simulink model "LorenzModel_book_example"  (R2023a)
settings: Solver=VariableStepAuto  StartTime=0.0  StopTime=50  RelTol=1e-3
settings Model: Creator=axobj  LastModifiedBy=axobj

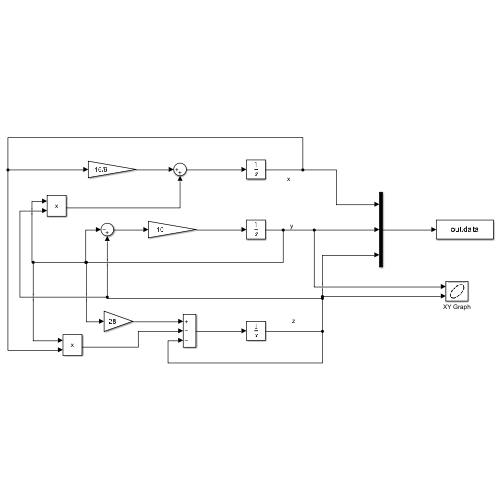
[thumbnail: Simulink's stored preview of the top-level diagram]
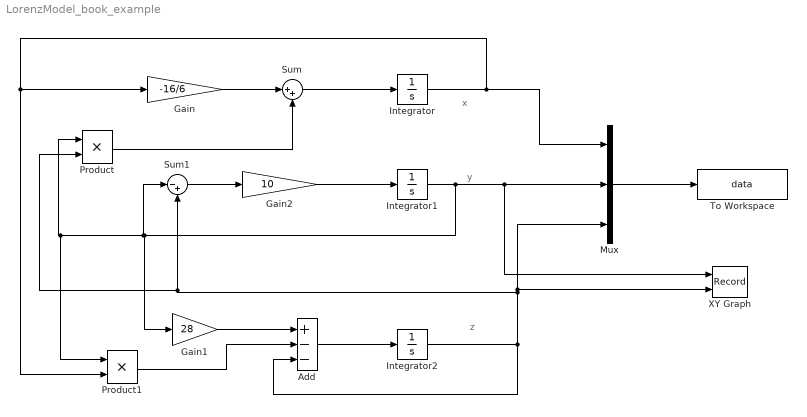
== system LorenzModel_book_example ==
  note: x
  note: y
  note: z
  Add : Sum  Inputs=+--
  Gain : Gain  Gain=-16/6
  Gain1 : Gain  Gain=28
  Gain2 : Gain  Gain=10
  Integrator : Integrator  InitialCondition=1
  Integrator1 : Integrator  InitialCondition=1
  Integrator2 : Integrator  InitialCondition=1
  Mux : Mux  Inputs=3
  Product : Product
  Product1 : Product
  Sum : Sum  Inputs=|++
  Sum1 : Sum  Inputs=|-+
  To Workspace : ToWorkspace  VariableName=data  SampleTime=-1
  XY Graph : Record  FileSettingsInternal="{\"entries\":[{\"content\":{\"excelSettings\":{\"content\":{},\"type\":\"Streamout.ExcelSettings\"}},\"type\":\"Streamout.FileSettingStorage\",\"uuid\":\"\"}],\"packageUris\":[\"http:\\/\\/schema.mathworks.com\\/mf0\\/streamout_blocks\\/R2020a\"],\"version\":\"1.0\"}"  Layout=[1 1]  SignalsInternal="{\"entries\":[{\"content\":{\"signals\":[{\"content\":{\"blockPath\":[],\"dimensions\":[1],\"domain\":\"\",\"lineColor\":\"#a2142f\",\"plots\":[1],\"port\":1,\"sid\":[\"\"],\"signalID\":522,\"signalName\":\"Integrator1\"},\"type\":\"RecordBlkView.Signal\",\"uuid\":\"\"},{\"content\":{\"blockPath\":[],\"dimensions\":[1],\"domain\":\"\",\"lineColor\":\"#139fff\",\"plots\":[1],\"port\":2,\"sid\":[\"\"],\"signalID\":526,\"signalName\":\"Integrator2\"},\"type\":\"RecordBlkView.Signal\",\"uuid\":\"\"}]},\"type\":\"RecordBlkView.InputSignals\",\"uuid\":\"\"}],\"packageUris\":[\"http:\\/\\/schema.mathworks.com\\/mf0\\/streamout_blocks\\/R2020a\"],\"version\":\"1.0\"}"  VisualizationBindings="{\"xyplotplugin\":{\"info\":[{\"series\":[{\"bindingParametersList\":[{\"parameter\":\"X-Axis\",\"signalID\":522,\"signalName\":\"Integrator1\"},{\"parameter\":\"Y-Axis\",\"signalID\":526,\"signalName\":\"Integrator2\"}],\"seriesID\":59284}],\"subplotID\":1}]}}"  CompatibilityTag=XY
  wires:
  Mux/1 -> To Workspace/1
  Integrator/1 -> Product1/2, Gain/1, Mux/1
  Integrator1/1 -> Product1/1, Product/1, Sum1/1, Gain1/1, XY Graph/1, Mux/2
  Integrator2/1 -> Add/3, XY Graph/2, Mux/3, Product/2, Sum1/2
  Sum1/1 -> Gain2/1
  Gain2/1 -> Integrator1/1
  Sum/1 -> Integrator/1
  Gain/1 -> Sum/1
  Product/1 -> Sum/2
  Add/1 -> Integrator2/1
  Gain1/1 -> Add/1
  Product1/1 -> Add/2
